simulink model "simulation"  (R2014a)
settings: Solver=ode45  StartTime=0.0  StopTime=10  RelTol=1e-3
libraries: simulink x1
settings Model: Creator=usmankhan  LastModifiedBy=usmankhan

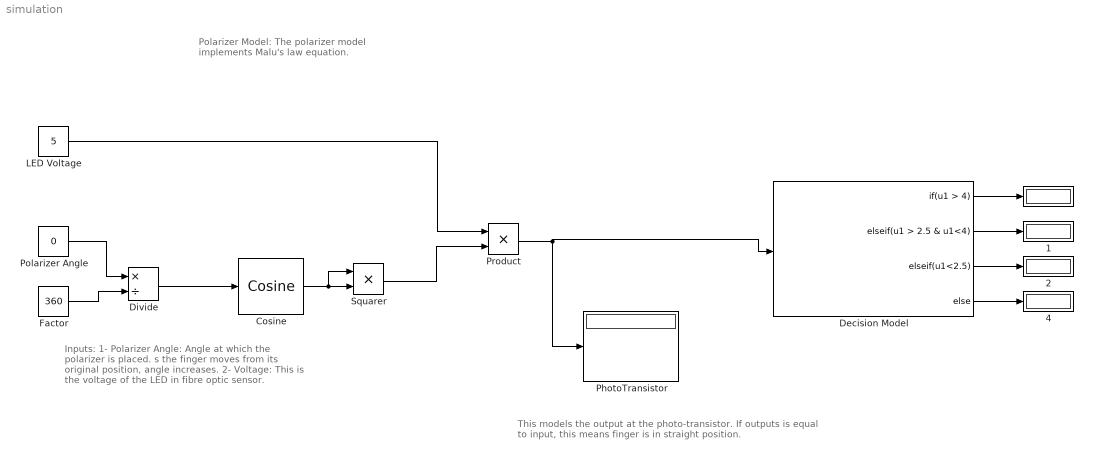
== system simulation ==
  note: Polarizer Model:
      |
      | The polarizer model implements
      | Malu's law equation.
  note: Inputs:
      |
      | 1- Polarizer Angle: Angle at which
      | the polarizer is placed. s the finger
      | moves from its original position, angle
      | increases.
      |
      | 2- Voltage: This is the voltage of the
      | LED in fibre optic sensor.
  note: This models the output at the photo-transistor.
      | If outputs is equal to input, this means finger
      | is in straight position.
   {,1..2,4} (4 alike) : Display
      settings: Format=binary (Stored Integer)
  " LED Voltage" : Constant  Value=5  SampleTime=Inf
  Cosine : simulink/Lookup Tables/Cosine  Formula=cos(2*pi*u)  NumDataPoints=(2^5)+1  OutputWordLength=16  InternalRulePriority=Speed
  Decision Model : If  IfExpression=u1 > 4  ElseIfExpressions=u1 > 2.5 & u1<4, u1<2.5  ZeroCross=off
  Divide : Product  Inputs=*/
  "Factor " : Constant  Value=360  SampleTime=Inf
  PhotoTransistor : Display
  Polarizer Angle : Constant  Value=0  SampleTime=Inf
  Product : Product
  Squarer : Product
  wires:
  Polarizer Angle/1 -> Divide/1
  Divide/1 -> Cosine/1
  "Factor "/1 -> Divide/2
  Cosine/1 -> Squarer/2, Squarer/1
  Squarer/1 -> Product/2
  " LED Voltage"/1 -> Product/1
  Product/1 -> PhotoTransistor/1, Decision Model/1
  Decision Model/1 -> " "/1
  Decision Model/4 -> " 4"/1
  Decision Model/3 -> " 2"/1
  Decision Model/2 -> " 1"/1
